simulink model "untitled"  (R2020b)
settings: Solver=VariableStepAuto  StartTime=0.0  StopTime=1500  MaxStep=1e-2  RelTol=1e-3
settings Model: Creator=Administrador  LastModifiedBy=Administrador

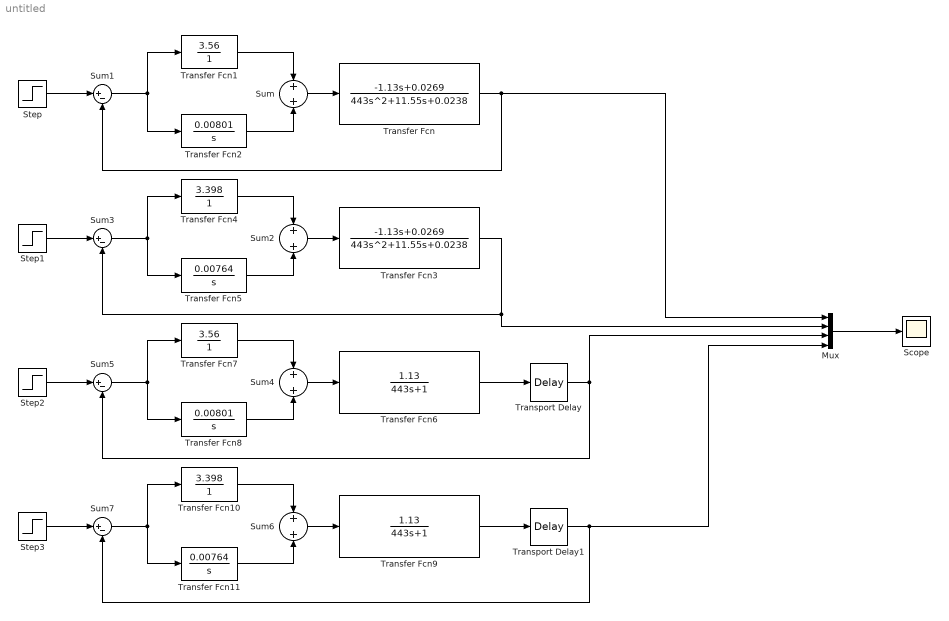
== system untitled ==
  Mux : Mux
  Scope : Scope
  Step{,1..3} (4 alike) : Step  Time=0  SampleTime=0
  Sum{,2,4,6} (4 alike) : Sum
  Sum{1,3,5,7} (4 alike) : Sum  Inputs=|+-
  Transfer Fcn : TransferFcn  Numerator=[-1.13 0.0269]  Denominator=[443 11.55 0.0238]
  Transfer Fcn1 : TransferFcn  Numerator=[3.56]  Denominator=[1]
  Transfer Fcn10 : TransferFcn  Numerator=[3.398]  Denominator=[1]
  Transfer Fcn11 : TransferFcn  Numerator=[0.00764]  Denominator=[1 0]
  Transfer Fcn2 : TransferFcn  Numerator=[0.00801]  Denominator=[1 0]
  Transfer Fcn3 : TransferFcn  Numerator=[-1.13 0.0269]  Denominator=[443 11.55 0.0238]
  Transfer Fcn4 : TransferFcn  Numerator=[3.398]  Denominator=[1]
  Transfer Fcn5 : TransferFcn  Numerator=[0.00764]  Denominator=[1 0]
  Transfer Fcn6 : TransferFcn  Numerator=[1.13]  Denominator=[443 1]
  Transfer Fcn7 : TransferFcn  Numerator=[3.56]  Denominator=[1]
  Transfer Fcn8 : TransferFcn  Numerator=[0.00801]  Denominator=[1 0]
  Transfer Fcn9 : TransferFcn  Numerator=[1.13]  Denominator=[443 1]
  Transport Delay : TransportDelay  DelayTime=84
  Transport Delay1 : TransportDelay  DelayTime=84
  wires:
  Transfer Fcn1/1 -> Sum/1
  Transfer Fcn2/1 -> Sum/2
  Sum1/1 -> Transfer Fcn1/1, Transfer Fcn2/1
  Sum/1 -> Transfer Fcn/1
  Step/1 -> Sum1/1
  Transfer Fcn/1 -> Mux/1, Sum1/2
  Transfer Fcn5/1 -> Sum2/2
  Sum2/1 -> Transfer Fcn3/1
  Step1/1 -> Sum3/1
  Transfer Fcn3/1 -> Mux/2, Sum3/2
  Transfer Fcn4/1 -> Sum2/1
  Sum3/1 -> Transfer Fcn4/1, Transfer Fcn5/1
  Sum5/1 -> Transfer Fcn7/1, Transfer Fcn8/1
  Transfer Fcn7/1 -> Sum4/1
  Sum4/1 -> Transfer Fcn6/1
  Transfer Fcn8/1 -> Sum4/2
  Step2/1 -> Sum5/1
  Transfer Fcn6/1 -> Transport Delay/1
  Transport Delay/1 -> Mux/3, Sum5/2
  Transfer Fcn11/1 -> Sum6/2
  Sum6/1 -> Transfer Fcn9/1
  Sum7/1 -> Transfer Fcn10/1, Transfer Fcn11/1
  Transfer Fcn10/1 -> Sum6/1
  Transfer Fcn9/1 -> Transport Delay1/1
  Transport Delay1/1 -> Mux/4, Sum7/2
  Step3/1 -> Sum7/1
  Mux/1 -> Scope/1
